simulink model "UAV_GCS_Base_Link"  (R2026a)
settings: Solver=FixedStepDiscrete  StopTime=0.01
libraries: commchan3 x1, commrandsrc3 x1
settings Model: Creator=Adi Suliman  LastModifiedBy=Adi Suliman

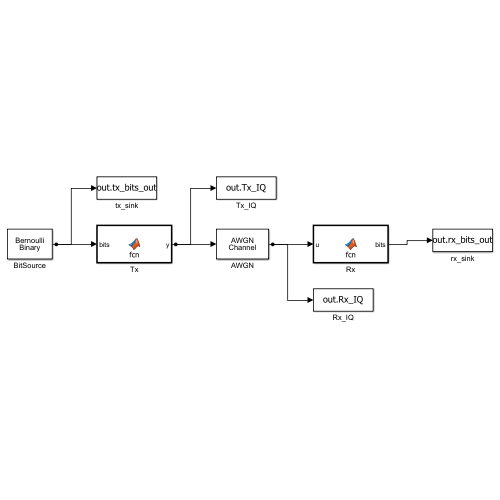
[thumbnail: Simulink's stored preview of the top-level diagram]
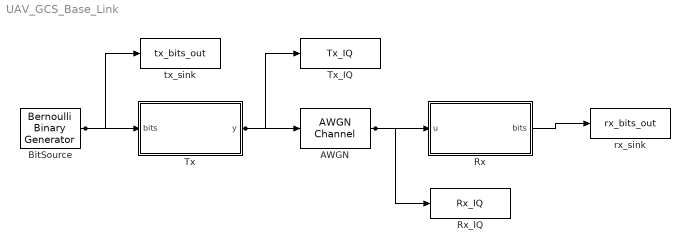
== system UAV_GCS_Base_Link ==
  AWGN : commchan3/AWGN Channel  LegacyMode=off  NoiseMethod="Signal to noise ratio  (SNR)"  noiseMode="Signal to noise ratio  (SNR)"  EbNo=10  EsNo=10  SNR=-3.0103  BitsPerSymbol=1  SignalPower=0.25  SpecifySymbolPeriod=off  SamplesPerSymbol=1  SymbolPeriod=1  VarianceSource=Parameter  Variance=1  RandomStream=Global stream  Seed=67  SimulateUsing=Code generation
  BitSource : commrandsrc3/Bernoulli Binary Generator  ProbabilityOfZero=0.5  SeedSource=Auto  Seed=0  SampleTime=5e-07  SamplesPerFrame=1032  OutputDataType=double  SimulateUsing=Interpreted execution
  Rx : MATLAB Function  TreatAsAtomicUnit=on
  Rx_IQ : ToWorkspace  VariableName=Rx_IQ  SampleTime=-1
  Tx : MATLAB Function  TreatAsAtomicUnit=on
  Tx_IQ : ToWorkspace  VariableName=Tx_IQ  SampleTime=-1
  rx_sink : ToWorkspace  VariableName=rx_bits_out  SampleTime=-1
  tx_sink : ToWorkspace  VariableName=tx_bits_out  SampleTime=-1
  wires:
  BitSource/1 -> Tx/1(bits), tx_sink/1
  Tx/1(y) -> AWGN/1, Tx_IQ/1
  AWGN/1 -> Rx/1(u), Rx_IQ/1
  Rx/1(bits) -> rx_sink/1

== matlab function UAV_GCS_Base_Link/Tx ==
  data: bits input; y output
function y = fcn(bits)
%#codegen
persistent txf
if isempty(txf)
    txf = comm.RaisedCosineTransmitFilter(...
        'RolloffFactor', 0.250000, ...
        'FilterSpanInSymbols', 10, ...
        'OutputSamplesPerSymbol', 4);
end
sym = pskmod(bits, 4, pi/4, 'gray', 'InputType', 'bit');
y = txf(sym);
end

== matlab function UAV_GCS_Base_Link/Rx ==
  data: u input; bits output
function bits = fcn(u)
%#codegen
persistent rxf
if isempty(rxf)
    rxf = comm.RaisedCosineReceiveFilter(...
        'RolloffFactor', 0.250000, ...
        'FilterSpanInSymbols', 10, ...
        'InputSamplesPerSymbol', 4, ...
        'DecimationFactor', 4);
end
sym = rxf(u);
bits = pskdemod(sym, 4, pi/4, 'gray', 'OutputType', 'bit');
end
